simulink model "datacapture_model"  (R2020b)
settings: Solver=VariableStepAuto  StartTime=0.0  StopTime=1023  RelTol=1e-3
libraries: hdlverifier_fpga_reader x1
settings Model: Creator=pablo  LastModifiedBy=pablo

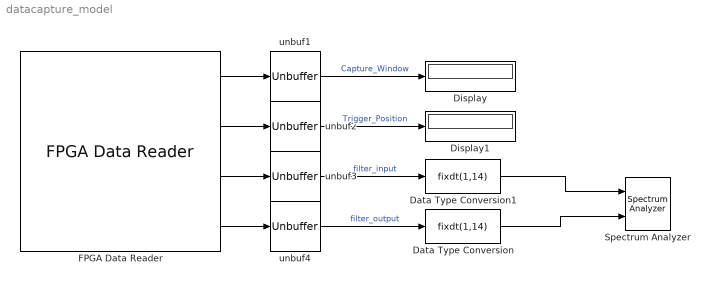
== system datacapture_model ==
  Data Type Conversion : DataTypeConversion  OutMin=-1  OutMax=1  OutDataTypeStr=fixdt(1,14)
  Data Type Conversion1 : DataTypeConversion  OutMin=-1  OutMax=1  OutDataTypeStr=fixdt(1,14)
  Display : Display
  Display1 : Display
  FPGA Data Reader : hdlverifier_fpga_reader/FPGA Data Reader  SampleTime=1024  FPGAVendor=Xilinx  SamplesPerFrame=1024  TriggerPosition=513  NumCaptureWindows=1  MaxNumTriggerStages=1  NumTriggerStages=1  TimeOut=10  TriggerConditionStr="[false,\"0\",\"==\",0,false,\"0\",\"==\",0,\"and\",0,1]"  DataTypeStr="[\"uint32\",\"boolean\",\"numerictype(0,14,0)\",\"numerictype(0,18,0)\"]"  BitWidth="[32   1  14  18]"  SignalNames={'Capture_Window','Trigger_Position','filter_input','filter_output'}  IsSignalTrigger="[0  0  1  1]"  IsSignalData="[0  0  1  1]"  IsMetaData="[1  1  0  0]"  RunImmediately=0  JTAGCableName=auto  JTAGCableType=auto  JTAGChainPosition=0  IRLengthBefore=0  IRLengthAfter=0  TckFrequency=15
      settings: SourceProductBaseCode=HDLVALTERA,INTEL_FPGA_SOC,XILINX_FPGA_SOC,INTEL_BLOCKSET,MICROSEMI,HDLCVXILINX,XILINX_BLOCKSET
  Spectrum Analyzer : SpectrumAnalyzer  NumInputPorts=2
  unbuf{1..4} (4 alike) : Unbuffer
  wires:
  FPGA Data Reader/1 -> unbuf1/1
  FPGA Data Reader/2 -> unbuf2/1
  FPGA Data Reader/3 -> unbuf3/1
  FPGA Data Reader/4 -> unbuf4/1
  unbuf4/1 -> Data Type Conversion/1  "filter_output"
  unbuf3/1 -> Data Type Conversion1/1  "filter_input"
  Data Type Conversion1/1 -> Spectrum Analyzer/1
  Data Type Conversion/1 -> Spectrum Analyzer/2
  unbuf1/1 -> Display/1  "Capture_Window"
  unbuf2/1 -> Display1/1  "Trigger_Position"
